simulink model "exercise13a"  (R2018b)
settings: Solver=VariableStepAuto  StartTime=0.0  StopTime=20  RelTol=1e-3
settings Model: Creator=Alireza  LastModifiedBy=Alireza

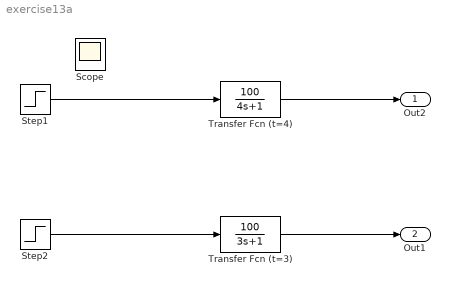
== system exercise13a ==
  Step1 : Step  SampleTime=0
  Step2 : Step  SampleTime=0
  Transfer Fcn (t=3) : TransferFcn  Numerator=[100]  Denominator=[3 1]
  Transfer Fcn (t=4) : TransferFcn  Numerator=[100]  Denominator=[4 1]
  Out2 : Outport
  Out1 : Outport  Port=2
  Scope : Scope
  wires:
  Transfer Fcn (t=3)/1 -> Out1/1
  Step1/1 -> Transfer Fcn (t=4)/1
  Step2/1 -> Transfer Fcn (t=3)/1
  Transfer Fcn (t=4)/1 -> Out2/1
